simulink model "fcn_test"  (R2017a)
settings: Solver=VariableStepAuto  StartTime=0.0  StopTime=10.0  RelTol=1e-3
settings Model: Creator=Instructor  LastModifiedBy=Instructor

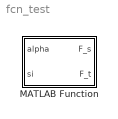
== system fcn_test ==
  MATLAB Function : MATLAB Function  TreatAsAtomicUnit=on

== matlab function fcn_test/MATLAB Function ==
  data: alpha input; F_s output; si input; F_t output
function [F_s,F_t] = fcn(alpha,si)

F_t = u;
